simulink model "Block_Diagram"  (R2025b)
settings: Solver=ode1  StartTime=0.0  StopTime=4  FixedStep=0.001  RelTol=1e-3
values from neighbouring files (symbols this model uses):
  a = ((R*f/r_m^2) + K_b*K_T*(r_g/r_m)^2) / (R*J/r_m^2 + R*M)    (= 10.9845986858)    [Main.m]
  b = (K_T*r_g*1/r_m) / (R*J/(r_m^2) + R*M)    (= 2.45125586982)    [Main.m]
  g = 9.81    [Main.m]
  K_D = R / (K_T*r_g/r_m)    (= 0.580200100507)    [Main.m]
  K_enc = 2.275*10^-5    (= 2.275e-05)    [Main.m]
  M = M_c    (= 0.57)    [Main.m]
  N_enc = 4*1024    (= 4096)    [Main.m]
  phi = 0    [Main.m]
  T = 0.001    [Main.m]
libraries: simulink x1
settings Model: Creator=arnes  LastModifiedBy=arnes
settings DataIOCC: Decimation=6

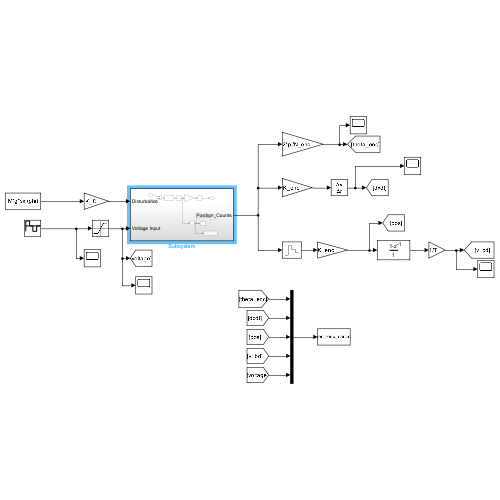
[thumbnail: Simulink's stored preview of the top-level diagram]
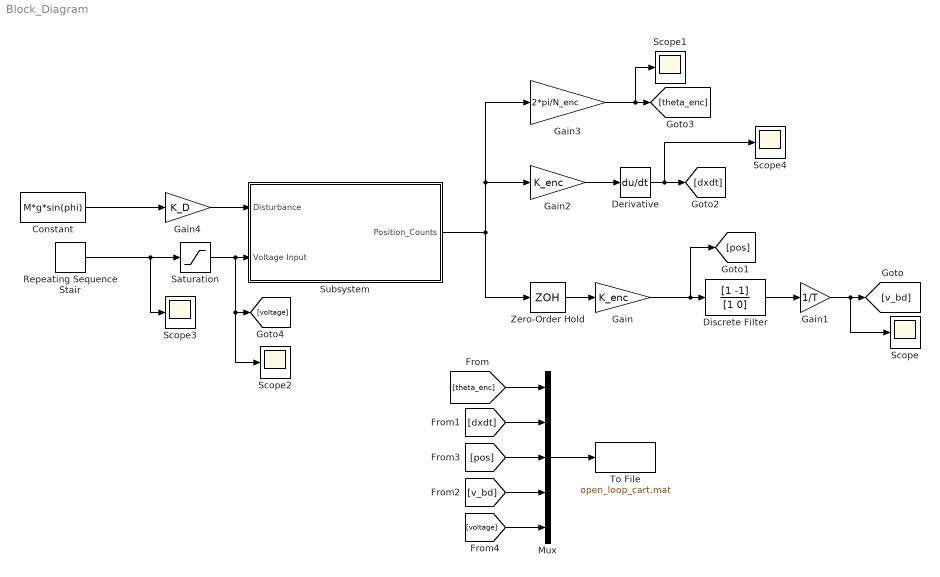
== system Block_Diagram ==
  Constant : Constant  Value=M*g*sin(phi)
  Derivative : Derivative
  Discrete Filter : DiscreteFilter  Numerator=[1 -1]  Denominator=[1 0]
  Gain : Gain  Gain=K_enc
  Gain1 : Gain  Gain=1/T
  Gain2 : Gain  Gain=K_enc
  Gain3 : Gain  Gain=2*pi/N_enc
  Gain4 : Gain  Gain=K_D
  Mux : Mux  Inputs=5
  Repeating Sequence Stair : simulink/Sources/Repeating Sequence Stair  OutValues=[2 00 -2 00].'  tsamp=1  OutMin=[]  OutMax=[]  OutDataTypeStr=double  OutputDataTypeScalingMode=double  OutDataType=fixdt(0,8)  ConRadixGroup=Best Precision: Vector-wise  OutScaling=2^-12
  Saturation : Saturate  UpperLimit=5  LowerLimit=-5
  Scope{,1..4} (5 alike) : Scope
      Scope settings: ActiveDisplayYMinimum=-0.56875000000004838  ActiveDisplayYMaximum=0.56875000000004838
      Scope1 settings: ActiveDisplayYMinimum=-3.761512639494077  ActiveDisplayYMaximum=33.8536137554467
      Scope2 settings: DataLoggingVariableName=ScopeData2
      Scope3 settings: DataLoggingVariableName=ScopeData3
      Scope4 settings: ActiveDisplayYMinimum=-0.0102099015988013  ActiveDisplayYMaximum=0.040798715828425321  DataLoggingVariableName=ScopeData4
  Subsystem : Subsystem
  To File : ToFile  Filename=open_loop_cart.mat  MatrixName=cart_data
  Zero-Order Hold : ZeroOrderHold  SampleTime=T
  wires:
  Gain/1 -> [pos], Discrete Filter/1
  Zero-Order Hold/1 -> Gain/1
  Discrete Filter/1 -> Gain1/1
  Gain1/1 -> Scope/1, [v_bd]
  Derivative/1 -> Scope4/1, [dxdt]
  Gain2/1 -> Derivative/1
  Gain3/1 -> Scope1/1, [theta_enc]
  Mux/1 -> To File/1
  [theta_enc] -> Mux/1
  [dxdt] -> Mux/2
  [pos] -> Mux/3
  [v_bd] -> Mux/4
  Subsystem/1(Position_Counts) -> Zero-Order Hold/1, Gain2/1, Gain3/1
  Saturation/1 -> Scope2/1, [voltage], Subsystem/2(Voltage Input)
  Gain4/1 -> Subsystem/1(Disturbance)
  [voltage] -> Mux/5
  Repeating Sequence Stair/1 -> Scope3/1, Saturation/1
  Constant/1 -> Gain4/1

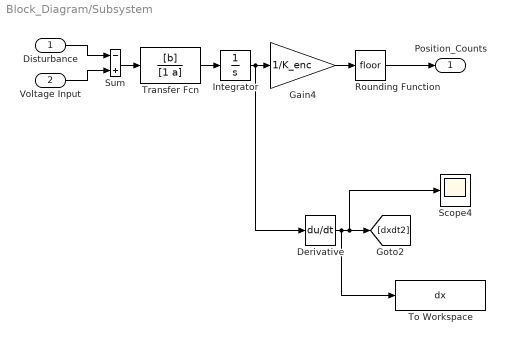
== system Block_Diagram/Subsystem ==
  Disturbance : Inport
  Voltage Input : Inport  Port=2
  Derivative : Derivative
  Gain4 : Gain  Gain=1/K_enc
  Integrator : Integrator
  Rounding Function : Rounding
  Scope4 : Scope
      settings: ActiveDisplayYMinimum=-0.098144858910795413  ActiveDisplayYMaximum=0.28660787034188773  DataLoggingVariableName=ScopeData5
  Sum : Sum  Inputs=-+
  To Workspace : ToWorkspace  VariableName=dx  SaveFormat=Timeseries  SampleTime=-1
  Transfer Fcn : TransferFcn  Numerator=[b]  Denominator=[1 a]
  Position_Counts : Outport
  wires:
  Sum/1 -> Transfer Fcn/1
  Disturbance/1 -> Sum/1
  Integrator/1 -> Derivative/1, Gain4/1
  Voltage Input/1 -> Sum/2
  Transfer Fcn/1 -> Integrator/1
  Rounding Function/1 -> Position_Counts/1
  Gain4/1 -> Rounding Function/1
  Derivative/1 -> To Workspace/1, Scope4/1, [dxdt2]
